simulink model "RackAndPinion"  (R2023a)
settings: Solver=VariableStepAuto  StartTime=0.0  StopTime=10.0  RelTol=1e-3
settings Model: Creator=ASUS TUF GAMING  LastModifiedBy=ASUS TUF GAMING

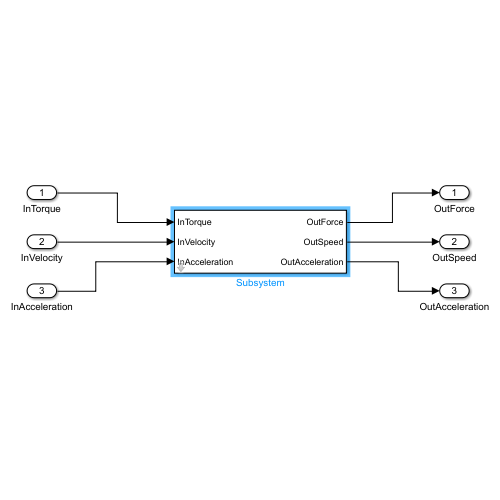
[thumbnail: Simulink's stored preview of the top-level diagram]
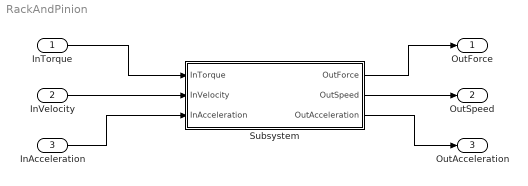
== system RackAndPinion ==
  InTorque : Inport
  InVelocity : Inport  Port=2
  InAcceleration : Inport  Port=3
  Subsystem : Subsystem  mask{i_gear=20, J_gear=1, vis_friction_coef_gear=0.001}
      mask prompts: i_gear "GeaGear aspect ratio, rad/mm"; J_gear "TheGear inertia, kg * m^2"; vis_friction_coef_gear "Viscous friction coefficient, kg * m^2 / s"
  OutForce : Outport
  OutSpeed : Outport  Port=2
  OutAcceleration : Outport  Port=3
  wires:
  InTorque/1 -> Subsystem/1(InTorque)
  InVelocity/1 -> Subsystem/2(InVelocity)
  InAcceleration/1 -> Subsystem/3(InAcceleration)
  Subsystem/1(OutForce) -> OutForce/1
  Subsystem/2(OutSpeed) -> OutSpeed/1
  Subsystem/3(OutAcceleration) -> OutAcceleration/1

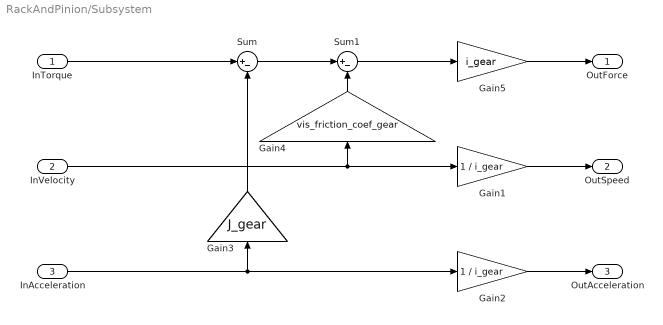
== system RackAndPinion/Subsystem ==
  InTorque : Inport
  InVelocity : Inport  Port=2
  InAcceleration : Inport  Port=3
  Gain1 : Gain  Gain=1 / i_gear
  Gain2 : Gain  Gain=1 / i_gear
  Gain3 : Gain  Gain=J_gear
  Gain4 : Gain  Gain=vis_friction_coef_gear
  Gain5 : Gain  Gain=i_gear
  Sum : Sum  Inputs=|+-
  Sum1 : Sum  Inputs=|+-
  OutForce : Outport
  OutSpeed : Outport  Port=2
  OutAcceleration : Outport  Port=3
  wires:
  InVelocity/1 -> Gain1/1, Gain4/1
  Gain1/1 -> OutSpeed/1
  InTorque/1 -> Sum/1
  Sum1/1 -> Gain5/1
  InAcceleration/1 -> Gain3/1, Gain2/1
  Gain2/1 -> OutAcceleration/1
  Gain4/1 -> Sum1/2
  Sum/1 -> Sum1/1
  Gain3/1 -> Sum/2
  Gain5/1 -> OutForce/1
